simulink model "Robot_moding"  (R2020b)
settings: Solver=VariableStepAuto  StartTime=0.0  StopTime=10.0  RelTol=1e-3
settings Model: Creator=60251  LastModifiedBy=60251

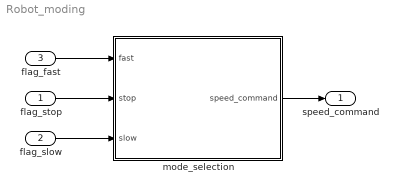
== system Robot_moding ==
  flag_stop : Inport
  flag_slow : Inport  Port=2
  flag_fast : Inport  Port=3
  mode_selection : Stateflow chart  TreatAsAtomicUnit=on
  speed_command : Outport
  wires:
  mode_selection/1(speed_command) -> speed_command/1
  flag_fast/1 -> mode_selection/1(fast)
  flag_slow/1 -> mode_selection/3(slow)
  flag_stop/1 -> mode_selection/2(stop)

== stateflow chart Robot_moding/mode_selection ==
  settings: stateMachineType=MEALY_MACHINE
  state Stop
  state Slow
  state Fast
  (default) -> Stop
  Stop -> Slow [order 1] : [slow == true]
      | {speed_command= 127;}
  Slow -> Fast [order 1] : [fast == true]
      | {speed_command = 255;}
  Slow -> Stop [order 2] : [stop == true]
      | {speed_command= 0;}
  Fast -> Slow [order 1] : [slow == true]
      | {speed_command= 127;}
  Fast -> Stop [order 2] : [stop == true]
      | {speed_command= 0;}
  Stop -> Fast [order 2] : [fast == true]
      | {speed_command= 255;}
  data: fast input boolean; stop input boolean; slow input boolean; speed_command output double
